simulink model "Crazyflie_CL_NL_Model"  (R2024a)
settings: Solver=ode23  StartTime=0.0  StopTime=Tend  FixedStep=dt  MaxStep=0.01  RelTol=1e-4
values from neighbouring files (symbols this model uses):
  ATTITUDE_RATE = 500    [crazyflie_Parameters.m]
  b = 1e-9    (= 1e-09)    [crazyflie_Parameters.m]
  cutoff_freq = 80    [crazyflie_Parameters.m]
  dt = 1/ATTITUDE_RATE    (= 0.002)    [crazyflie_Parameters.m]
  eta_eq0 = [0;0;0]    [Equilibrium_point.m]
  eta_init = eta_eq0    [Equilibrium_point.m]
  grav = 9.81    [crazyflie_Parameters.m]
  haero = 0    [crazyflie_Parameters.m]
  Jxx = rho_x_y*a_side*height*(a_side^2+height^2)/12    [crazyflie_Parameters.m]
  Jyy = rho_x_y*a_side*height*(a_side^2+height^2)/12    [crazyflie_Parameters.m]
  Jzz = rho_z*a_side^4/6    [crazyflie_Parameters.m]
  K = blkdiag(Kroll,Kpitch,Kyaw)*[1 0 0 0 0 0 ... (first row only)    [Basic_Classical_FR_control_design.m]
  kconst = 1.95e-8    (= 1.95e-08)    [crazyflie_Parameters.m]
  L = sqrt(a_side^2+a_side^2)/2    [crazyflie_Parameters.m]
  masse = 29e-3    (= 0.029)    [crazyflie_Parameters.m]
  MAXINT16 = 2^16-1    (= 65535)    [crazyflie_Parameters.m]
  Mc2u = [1  -0.5  0.5 -1 ... (first row only)    [crazyflie_Parameters.m]
  muxy = 0.4*masse    (= 0.0116)    [crazyflie_Parameters.m]
  muz = 5e-2    (= 0.05)    [crazyflie_Parameters.m]
  p0 = 280.93    [crazyflie_Parameters.m]
  p1 = 719.86    [crazyflie_Parameters.m]
  p2 = -15.689    [crazyflie_Parameters.m]
  p3 = 0.19157    [crazyflie_Parameters.m]
  p4 = -0.00082934    [crazyflie_Parameters.m]
  pdot_init = pdot_eq0    [Equilibrium_point.m]
  pitchSP = 2    [Equilibrium_point.m]
  pitchSPtime = 3    [Equilibrium_point.m]
  rollSP = 4    [Equilibrium_point.m]
  rollSPtime = 2.5    [Equilibrium_point.m]
  thurstSP = Tc    [Equilibrium_point.m]
  up = inpts(3)    [Equilibrium_point.m]    (also in mi_dron_film.m = R*[0;0;1])
  ur = inpts(2)    [Equilibrium_point.m]
  uy = inpts(4)    [Equilibrium_point.m]
  w_eq0 = [0;0;0]    [Equilibrium_point.m]
  w_init = w_eq0    [Equilibrium_point.m]
  yawSP = -3    [Equilibrium_point.m]
  yawSPtime = 2.1    [Equilibrium_point.m]
libraries: dspfdesign x6, cstblocks x1
settings Model: Creator=JB255047  LastModifiedBy=anton
settings SolverCC: AlgebraicLoopSolver=TrustRegion  DecoupledContinuousIntegration=on
settings DataIOCC: LimitDataPoints=on  SaveOutput=off  SignalLogging=off  DSMLogging=off  SaveTime=off
settings OptimizationCC: ExpressionDepthLimit=2147483647  LifeSpan=1
settings DebuggingCC: UnderspecifiedInitializationDetection=Classic  MergeDetectMultiDrivingBlocksExec=none  MultiTaskDSMMsg=none  FcnCallInpInsideContextMsg=warning  UnconnectedInputMsg=warning  UnconnectedOutputMsg=warning  UnconnectedLineMsg=warning  AllowSymbolicDim=off  StateNameClashWarn=warning  StrictBusMsg=ErrorOnBusTreatedAsVector  SFUnexpectedBacktrackingDiag=warning  SFNoUnconditionalDefaultTransitionDiag=warning  SFExecutionAtInitializationDiag=none  ArithmeticOperatorsInVariantConditions=warning
settings ModelReferenceCC: UpdateModelReferenceTargets=IfOutOfDate  EnableRefExpFcnMdlSchedulingChecks=on
settings SFSimCC: SFSimEcho=off  SimUseLocalCustomCode=off  CustomCodeUndefinedFunction=UseInterfaceOnly
settings RTWCC: RTWUseLocalCustomCode=off  GPUComputeCapability=3.5  DLArmComputeVersion=19.05
settings CodeAppCC: StateflowObjectComments=on
settings GRTTargetCC: TargetLangStandard=C89/C90 (ANSI)  CombineOutputUpdateFcns=off  GRTInterface=on

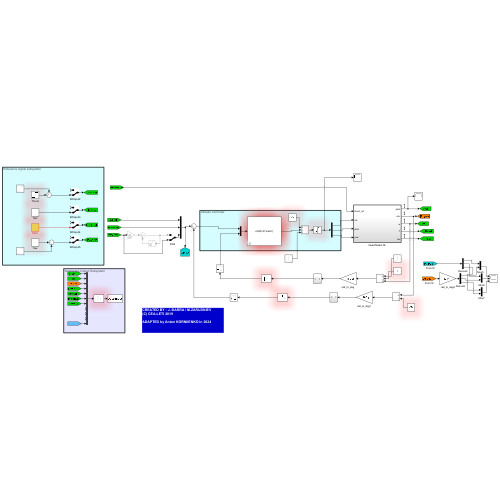
[thumbnail: Simulink's stored preview of the top-level diagram]
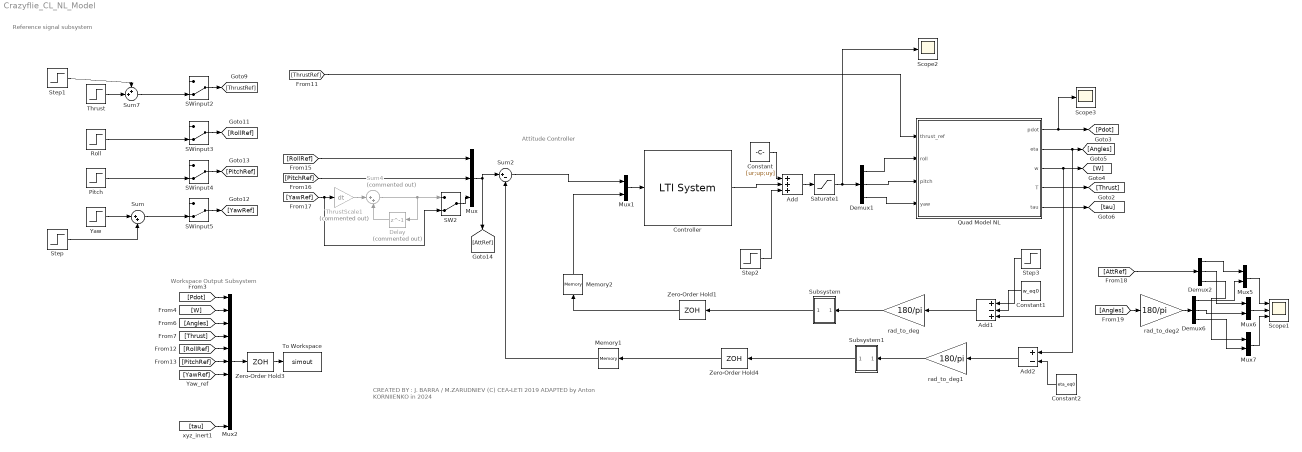
== system Crazyflie_CL_NL_Model ==
  note: CREATED BY : J. BARRA / M.ZARUDNIEV
      | (C) CEA-LETI 2019
      |
      | ADAPTED by Anton KORNIIENKO in 2024
  note: Workspace Output Subsystem
  note: Reference signal subsystem
  note: Attitude Controller
  Add : Sum  Inputs=+++
  Add1 : Sum  Inputs=+-+
  Add2 : Sum  Inputs=+-
  Constant : Constant  Value=[ur;up;uy]
  Constant1 : Constant  Value=w_eq0
  Constant2 : Constant  Value=eta_eq0
  Controller : cstblocks/LTI System  sys=c2d(K,dt,'tustin')  IC=[]  PadeOrder=0
  Delay : Delay  Commented=on  DelayLength=1  SampleTime=dt
  Demux1 : Demux  Outputs=3
  Demux2 : Demux  Outputs=3
  Demux6 : Demux  Outputs=3
  Memory1 : Memory
  Memory2 : Memory
  Mux : Mux  Inputs=3
  Mux{1,5..7} (4 alike) : Mux  Inputs=2
  Mux2 : Mux  Inputs=11
  Pitch : Step  Time=pitchSPtime  Before=up  After=pitchSP  SampleTime=0
  Quad Model NL : Subsystem  TreatAsAtomicUnit=on
  Roll : Step  Time=rollSPtime  Before=ur  After=rollSP  SampleTime=0
  SW2 : ManualSwitch  CurrentSetting=0
  SWinput{2..5} (4 alike) : ManualSwitch  CurrentSetting=0
  Saturate1 : Saturate  UpperLimit=MAXINT16/2-1  LowerLimit=-MAXINT16/2
  Scope1 : Scope  NumInputPorts=3
  Scope2 : Scope
  Scope3 : Scope
  Step : Step  Time=6.2  After=0  SampleTime=0
  Step1 : Step  Time=5  After=10000  SampleTime=0
  Step2 : Step  Time=7  After=-1000  SampleTime=0
  Step3 : Step  Time=14  SampleTime=0
  Subsystem : Subsystem
  Subsystem1 : Subsystem
  Sum : Sum  Inputs=|++
  Sum2 : Sum  Inputs=|+-
  Sum4 : Sum  Commented=on  Inputs=|++
  Sum7 : Sum  Inputs=++|
  Thrust : Step  Time=0  After=thurstSP  SampleTime=0
  ThrustScale1 : Gain  Commented=on  Gain=dt
  To Workspace : ToWorkspace  VariableName=simout  SaveFormat=Timeseries  SampleTime=-1
  Yaw : Step  Time=yawSPtime  Before=uy  After=yawSP  SampleTime=0
  Zero-Order Hold1 : ZeroOrderHold  SampleTime=1/ATTITUDE_RATE
  Zero-Order Hold3 : ZeroOrderHold  SampleTime=dt
  Zero-Order Hold4 : ZeroOrderHold  SampleTime=1/ATTITUDE_RATE
  rad_to_deg : Gain  Gain=180/pi
  rad_to_deg1 : Gain  Gain=180/pi
  rad_to_deg2 : Gain  Gain=180/pi
  wires:
  Sum2/1 -> Mux1/1
  Mux/1 -> Sum2/1, [AttRef]
  [ThrustRef] -> Quad Model NL/1(thrust_ref)
  Quad Model NL/3(w) -> Add1/3, [W]
  Mux2/1 -> Zero-Order Hold3/1
  Zero-Order Hold3/1 -> To Workspace/1
  [RollRef] -> Mux2/5
  [Pdot] -> Mux2/1
  [W] -> Mux2/2
  SWinput2/1 -> [ThrustRef]
  SWinput3/1 -> [RollRef]
  SWinput4/1 -> [PitchRef]
  SWinput5/1 -> [YawRef]
  Delay/1 -> Sum4/2
  [YawRef] -> SW2/2, ThrustScale1/1
  ThrustScale1/1 -> Sum4/1
  Sum4/1 -> SW2/1, Delay/1
  [PitchRef] -> Mux/2
  [RollRef] -> Mux/1
  Zero-Order Hold1/1 -> Memory2/1
  Zero-Order Hold4/1 -> Memory1/1
  Quad Model NL/2("eta ") -> Add2/1, [Angles]
  Memory1/1 -> Sum2/2
  Demux2/2 -> Mux6/1
  Demux6/2 -> Mux6/2
  Mux7/1 -> Scope1/3
  Mux6/1 -> Scope1/2
  Mux5/1 -> Scope1/1
  Demux2/3 -> Mux7/1
  Demux6/3 -> Mux7/2
  [AttRef] -> Demux2/1
  Demux6/1 -> Mux5/2
  Demux2/1 -> Mux5/1
  [Angles] -> rad_to_deg2/1
  SW2/1 -> Mux/3
  Roll/1 -> SWinput3/2
  Pitch/1 -> SWinput4/2
  Yaw/1 -> Sum/1
  Sum/1 -> SWinput5/2
  Step/1 -> Sum/2
  Quad Model NL/1(pdot) -> Scope3/1, [Pdot]
  Sum7/1 -> SWinput2/2
  Thrust/1 -> Sum7/2
  Step1/1 -> Sum7/1
  [Angles] -> Mux2/3
  [Thrust] -> Mux2/4
  [PitchRef] -> Mux2/6
  [YawRef] -> Mux2/7
  Quad Model NL/4(T) -> [Thrust]
  Quad Model NL/5(tau) -> [tau]
  [tau] -> Mux2/11
  rad_to_deg1/1 -> Subsystem1/1(In1)
  rad_to_deg/1 -> Subsystem/1(In1)
  Subsystem/1(Out1) -> Zero-Order Hold1/1
  Subsystem1/1(Out1) -> Zero-Order Hold4/1
  rad_to_deg2/1 -> Demux6/1
  Memory2/1 -> Mux1/2
  Mux1/1 -> Controller/1
  Demux1/1 -> Quad Model NL/2(roll)
  Demux1/2 -> Quad Model NL/3(pitch)
  Demux1/3 -> Quad Model NL/4(yaw)
  Add/1 -> Saturate1/1
  Constant/1 -> Add/1
  Controller/1 -> Add/2
  Saturate1/1 -> Scope2/1, Demux1/1
  Add1/1 -> rad_to_deg/1
  Add2/1 -> rad_to_deg1/1
  Constant1/1 -> Add1/2
  Constant2/1 -> Add2/2
  Step2/1 -> Add/3
  Step3/1 -> Add1/1

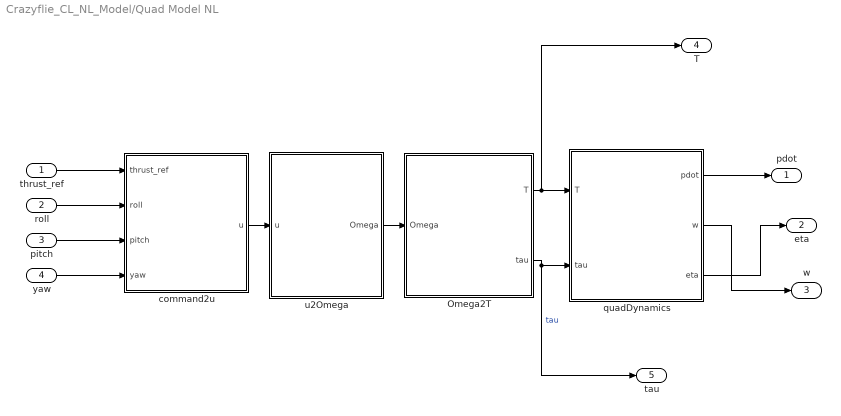
== system Crazyflie_CL_NL_Model/Quad Model NL ==
  thrust_ref : Inport
  roll : Inport  Port=2
  pitch : Inport  Port=3
  yaw : Inport  Port=4
  Omega2T : Subsystem  InitFcn=Omega=zeros(4,1);
  command2u : Subsystem  InitFcn=u=zeros(4,1);
  "quadDynamics " : Subsystem
  u2Omega : Subsystem
  pdot : Outport  VectorParamsAs1DForOutWhenUnconnected=off
  "eta " : Outport  Port=2  VectorParamsAs1DForOutWhenUnconnected=off
  w : Outport  Port=3  VectorParamsAs1DForOutWhenUnconnected=off
  T : Outport  Port=4  VectorParamsAs1DForOutWhenUnconnected=off
  tau : Outport  Port=5  VectorParamsAs1DForOutWhenUnconnected=off
  wires:
  "quadDynamics "/2(w) -> w/1
  "quadDynamics "/1(pdot) -> pdot/1
  "quadDynamics "/3(eta) -> "eta "/1
  Omega2T/1(T) -> "quadDynamics "/1(T), T/1
  thrust_ref/1 -> command2u/1(thrust_ref)
  roll/1 -> command2u/2(roll)
  pitch/1 -> command2u/3(pitch)
  yaw/1 -> command2u/4(yaw)
  Omega2T/2(tau) -> "quadDynamics "/2(tau), tau/1  "tau"
  u2Omega/1(Omega) -> Omega2T/1(Omega)
  command2u/1(u) -> u2Omega/1(u)

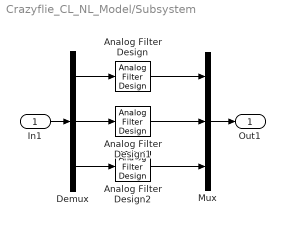
== system Crazyflie_CL_NL_Model/Subsystem ==
  In1 : Inport
  Analog Filter Design : dspfdesign/Analog Filter Design  method=Butterworth  filttype=Lowpass  N=2  Wlo=2*pi*cutoff_freq  Whi=80  Rp=2  Rs=40
  Analog Filter Design1 : dspfdesign/Analog Filter Design  method=Butterworth  filttype=Lowpass  N=2  Wlo=2*pi*cutoff_freq  Whi=80  Rp=2  Rs=40
  Analog Filter Design2 : dspfdesign/Analog Filter Design  method=Butterworth  filttype=Lowpass  N=2  Wlo=2*pi*cutoff_freq  Whi=80  Rp=2  Rs=40
  Demux : Demux  Outputs=3
  Mux : Mux  Inputs=3
  Out1 : Outport  VectorParamsAs1DForOutWhenUnconnected=off
  wires:
  In1/1 -> Demux/1
  Demux/1 -> Analog Filter Design/1
  Demux/2 -> Analog Filter Design1/1
  Demux/3 -> Analog Filter Design2/1
  Analog Filter Design1/1 -> Mux/2
  Analog Filter Design/1 -> Mux/1
  Analog Filter Design2/1 -> Mux/3
  Mux/1 -> Out1/1

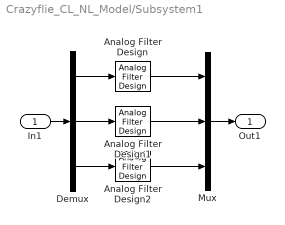
== system Crazyflie_CL_NL_Model/Subsystem1 ==
  In1 : Inport
  Analog Filter Design : dspfdesign/Analog Filter Design  method=Butterworth  filttype=Lowpass  N=2  Wlo=2*pi*cutoff_freq  Whi=80  Rp=2  Rs=40
  Analog Filter Design1 : dspfdesign/Analog Filter Design  method=Butterworth  filttype=Lowpass  N=2  Wlo=2*pi*cutoff_freq  Whi=80  Rp=2  Rs=40
  Analog Filter Design2 : dspfdesign/Analog Filter Design  method=Butterworth  filttype=Lowpass  N=2  Wlo=2*pi*cutoff_freq  Whi=80  Rp=2  Rs=40
  Demux : Demux  Outputs=3
  Mux : Mux  Inputs=3
  Out1 : Outport  VectorParamsAs1DForOutWhenUnconnected=off
  wires:
  In1/1 -> Demux/1
  Demux/1 -> Analog Filter Design/1
  Demux/2 -> Analog Filter Design1/1
  Demux/3 -> Analog Filter Design2/1
  Analog Filter Design1/1 -> Mux/2
  Analog Filter Design/1 -> Mux/1
  Analog Filter Design2/1 -> Mux/3
  Mux/1 -> Out1/1

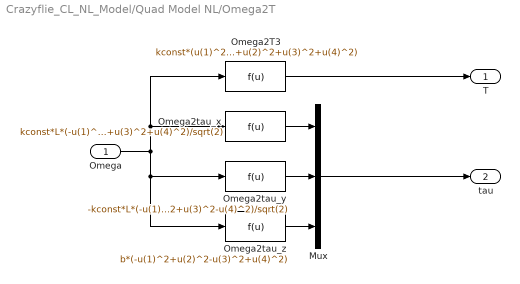
== system Crazyflie_CL_NL_Model/Quad Model NL/Omega2T ==
  Omega : Inport  PortDimensions=4
  Mux : Mux  Inputs=3
  Omega2T3 : Fcn  Expr=kconst*(u(1)^2+u(2)^2+u(3)^2+u(4)^2)
  Omega2tau_x : Fcn  Expr=kconst*L*(-u(1)^2-u(2)^2+u(3)^2+u(4)^2)/sqrt(2)
  Omega2tau_y : Fcn  Expr=-kconst*L*(-u(1)^2+u(2)^2+u(3)^2-u(4)^2)/sqrt(2)
  Omega2tau_z : Fcn  Expr=b*(-u(1)^2+u(2)^2-u(3)^2+u(4)^2)
  T : Outport  VectorParamsAs1DForOutWhenUnconnected=off
  tau : Outport  Port=2  VectorParamsAs1DForOutWhenUnconnected=off
  wires:
  Omega/1 -> Omega2T3/1, Omega2tau_x/1, Omega2tau_y/1, Omega2tau_z/1
  Omega2tau_z/1 -> Mux/3
  Omega2tau_x/1 -> Mux/1
  Omega2tau_y/1 -> Mux/2
  Mux/1 -> tau/1
  Omega2T3/1 -> T/1

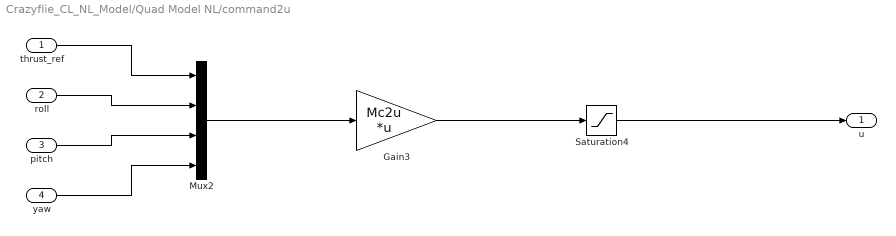
== system Crazyflie_CL_NL_Model/Quad Model NL/command2u ==
  thrust_ref : Inport
  roll : Inport  Port=2
  pitch : Inport  Port=3
  yaw : Inport  Port=4
  Gain3 : Gain  Gain=Mc2u  Multiplication=Matrix(K*u)
  Mux2 : Mux
  Saturation4 : Saturate  UpperLimit=MAXINT16  LowerLimit=0  LinearizeAsGain=off  ZeroCross=off
  u : Outport  VectorParamsAs1DForOutWhenUnconnected=off
  wires:
  thrust_ref/1 -> Mux2/1
  roll/1 -> Mux2/2
  pitch/1 -> Mux2/3
  yaw/1 -> Mux2/4
  Mux2/1 -> Gain3/1
  Gain3/1 -> Saturation4/1
  Saturation4/1 -> u/1

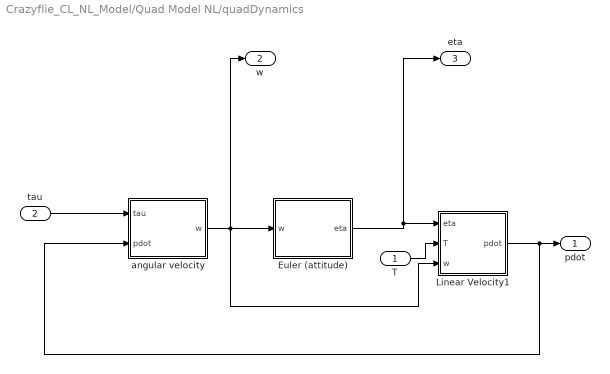
== system Crazyflie_CL_NL_Model/Quad Model NL/quadDynamics  ==
  T : Inport
  tau : Inport  Port=2
  "Euler (attitude) " : Subsystem
  Linear Velocity1 : Subsystem
  angular velocity : Subsystem
  pdot : Outport  PortDimensions=3  VectorParamsAs1DForOutWhenUnconnected=off
  w : Outport  Port=2  PortDimensions=3  VectorParamsAs1DForOutWhenUnconnected=off
  eta : Outport  Port=3  PortDimensions=3  VectorParamsAs1DForOutWhenUnconnected=off
  wires:
  T/1 -> Linear Velocity1/2(T)
  Linear Velocity1/1(pdot) -> angular velocity/2(pdot), pdot/1
  tau/1 -> angular velocity/1(tau)
  "Euler (attitude) "/1("eta ") -> eta/1, Linear Velocity1/1(eta)
  angular velocity/1(w) -> Linear Velocity1/3(w), w/1, "Euler (attitude) "/1(w)

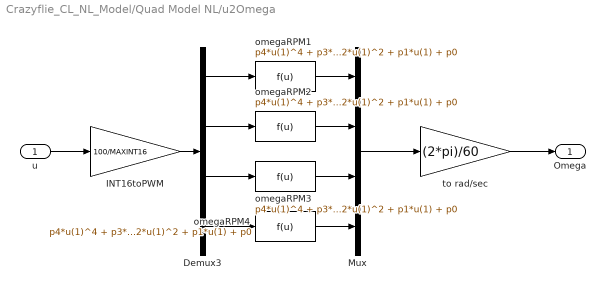
== system Crazyflie_CL_NL_Model/Quad Model NL/u2Omega ==
  u : Inport  PortDimensions=4
  Demux3 : Demux
  INT16toPWM : Gain  Gain=100/MAXINT16
  Mux : Mux
  omegaRPM{1..4} (4 alike) : Fcn  Expr=p4*u(1)^4 + p3*u(1)^3 + p2*u(1)^2 + p1*u(1) + p0
  to rad/sec : Gain  Gain=(2*pi)/60
  Omega : Outport  PortDimensions=4  VectorParamsAs1DForOutWhenUnconnected=off
  wires:
  u/1 -> INT16toPWM/1
  Mux/1 -> to rad/sec/1
  INT16toPWM/1 -> Demux3/1
  omegaRPM1/1 -> Mux/1
  Demux3/1 -> omegaRPM1/1
  Demux3/2 -> omegaRPM2/1
  omegaRPM2/1 -> Mux/2
  Demux3/3 -> omegaRPM3/1
  Demux3/4 -> omegaRPM4/1
  omegaRPM3/1 -> Mux/3
  omegaRPM4/1 -> Mux/4
  to rad/sec/1 -> Omega/1

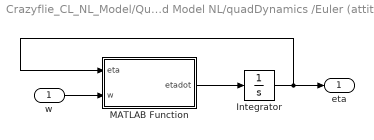
== system Crazyflie_CL_NL_Model/Quad Model NL/quadDynamics /Euler (attitude)  ==
  w : Inport  OutDataTypeStr=double
  Integrator : Integrator  InitialCondition=eta_init
  MATLAB Function : MATLAB Function  TreatAsAtomicUnit=on
  "eta " : Outport  VectorParamsAs1DForOutWhenUnconnected=off
  wires:
  Integrator/1 -> MATLAB Function/1(eta), "eta "/1
  w/1 -> MATLAB Function/2(w)
  MATLAB Function/1(etadot) -> Integrator/1

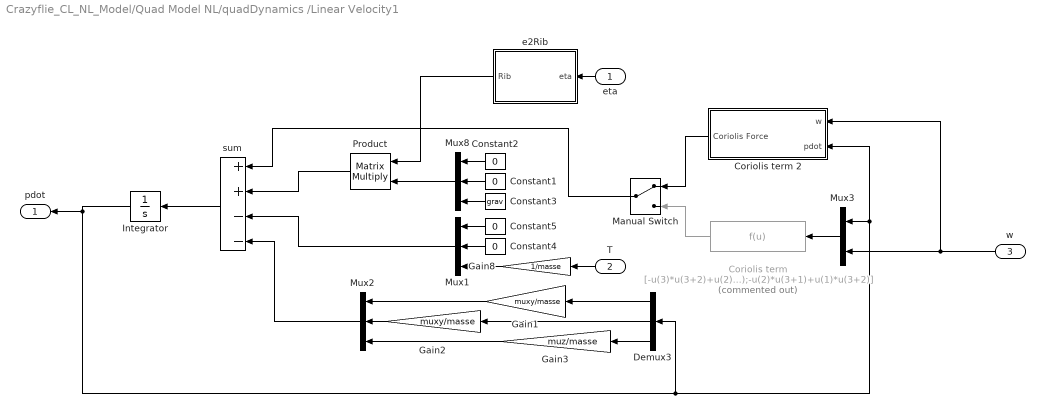
== system Crazyflie_CL_NL_Model/Quad Model NL/quadDynamics /Linear Velocity1 ==
  eta : Inport
  T : Inport  Port=2
  w : Inport  Port=3
  Constant{1..2,4..5} (4 alike) : Constant  Value=0
  Constant3 : Constant  Value=grav
  Coriolis term : Fcn  Commented=on  Expr=[-u(3)*u(3+2)+u(2)*u(3+3);-u(1)*u(3+3)+u(3)*u(3+1);-u(2)*u(3+1)+u(1)*u(3+2)]
  Coriolis term 2 : Subsystem
  Demux3 : Demux  Outputs=3
  Gain1 : Gain  Gain=muxy/masse
  Gain2 : Gain  Gain=muxy/masse
  Gain3 : Gain  Gain=muz/masse
  Gain8 : Gain  Gain=1/masse
  Integrator : Integrator  InitialCondition=pdot_init
  Manual Switch : ManualSwitch
  Mux1 : Mux  Inputs=3
  Mux2 : Mux  Inputs=3
  Mux3 : Mux  Inputs=2
  Mux8 : Mux  Inputs=3
  Product : Product  Multiplication=Matrix(*)  InputSameDT=on  SaturateOnIntegerOverflow=on  OutDataTypeStr=Inherit: Same as first input
  e2Rib : Subsystem
  sum : Sum  Inputs=++--
  pdot : Outport  PortDimensions=3  VectorParamsAs1DForOutWhenUnconnected=off
  wires:
  Constant1/1 -> Mux8/2
  Integrator/1 -> Demux3/1, Coriolis term 2/2(pdot), Mux3/1, pdot/1
  Constant4/1 -> Mux1/2
  T/1 -> Gain8/1
  Constant5/1 -> Mux1/1
  Gain1/1 -> Mux2/1
  Gain3/1 -> Mux2/3
  Gain8/1 -> Mux1/3
  Demux3/3 -> Gain3/1
  Gain2/1 -> Mux2/2
  eta/1 -> e2Rib/1(eta)
  Constant2/1 -> Mux8/1
  Mux2/1 -> sum/4
  sum/1 -> Integrator/1
  Mux1/1 -> sum/3
  Product/1 -> sum/2
  Constant3/1 -> Mux8/3
  Mux8/1 -> Product/2
  Demux3/1 -> Gain1/1
  Demux3/2 -> Gain2/1
  e2Rib/1(Rib) -> Product/1
  w/1 -> Coriolis term 2/1(w), Mux3/2
  Mux3/1 -> Coriolis term/1
  Coriolis term/1 -> Manual Switch/2
  Manual Switch/1 -> sum/1
  Coriolis term 2/1(Coriolis Force) -> Manual Switch/1

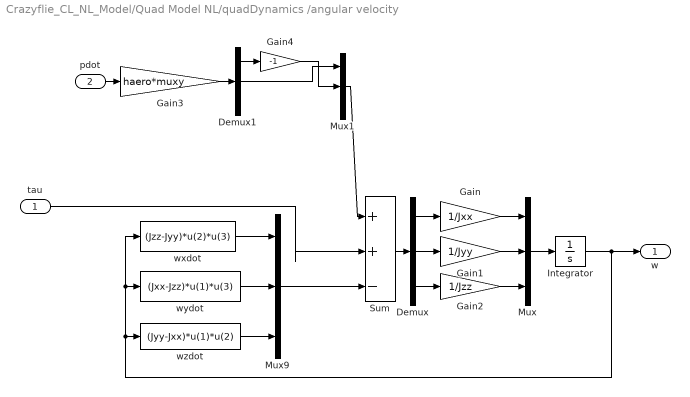
== system Crazyflie_CL_NL_Model/Quad Model NL/quadDynamics /angular velocity ==
  tau : Inport
  pdot : Inport  Port=2
  Demux : Demux  Outputs=3
  Demux1 : Demux  Outputs=3
  Gain : Gain  Gain=1/Jxx
  Gain1 : Gain  Gain=1/Jyy
  Gain2 : Gain  Gain=1/Jzz
  Gain3 : Gain  Gain=haero*muxy
  Gain4 : Gain  Gain=-1
  Integrator : Integrator  InitialCondition=w_init
  Mux : Mux  Inputs=3
  Mux1 : Mux  Inputs=3
  Mux9 : Mux  Inputs=3
  Sum : Sum  Inputs=|++-
  wxdot : Fcn  Expr=(Jzz-Jyy)*u(2)*u(3)
  wydot : Fcn  Expr=(Jxx-Jzz)*u(1)*u(3)
  wzdot : Fcn  Expr=(Jyy-Jxx)*u(1)*u(2)
  w : Outport  PortDimensions=3  VectorParamsAs1DForOutWhenUnconnected=off
  wires:
  wzdot/1 -> Mux9/3
  Sum/1 -> Demux/1
  Demux/1 -> Gain/1
  Demux/2 -> Gain1/1
  Demux/3 -> Gain2/1
  Gain/1 -> Mux/1
  Gain1/1 -> Mux/2
  Gain2/1 -> Mux/3
  Mux/1 -> Integrator/1
  Integrator/1 -> w/1, wzdot/1, wydot/1, wxdot/1
  wydot/1 -> Mux9/2
  wxdot/1 -> Mux9/1
  pdot/1 -> Gain3/1
  Gain3/1 -> Demux1/1
  Demux1/2 -> Mux1/1
  Mux1/1 -> Sum/1
  Demux1/1 -> Gain4/1
  Gain4/1 -> Mux1/2
  tau/1 -> Sum/2
  Mux9/1 -> Sum/3

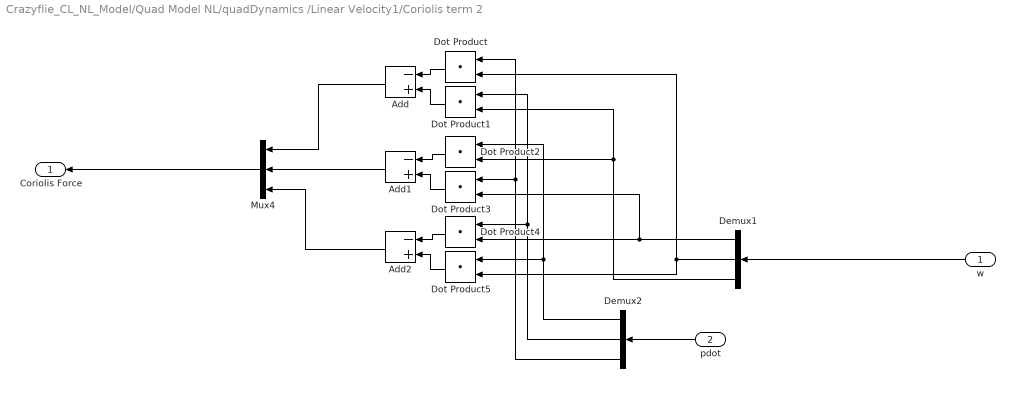
== system Crazyflie_CL_NL_Model/Quad Model NL/quadDynamics /Linear Velocity1/Coriolis term 2 ==
  w : Inport
  pdot : Inport  Port=2
  Add : Sum  Inputs=-+
  Add1 : Sum  Inputs=-+
  Add2 : Sum  Inputs=-+
  Demux1 : Demux  Outputs=3
  Demux2 : Demux  Outputs=3
  Dot Product{,1..5} (6 alike) : DotProduct  OutDataTypeStr=Inherit: Inherit via internal rule
  Mux4 : Mux  Inputs=3
  Coriolis Force : Outport
  wires:
  Demux2/1 -> Dot Product5/1, Dot Product2/1
  Add/1 -> Mux4/1
  Dot Product4/1 -> Add2/1
  Demux1/1 -> Dot Product4/2, Dot Product3/2
  Dot Product1/1 -> Add/2
  Demux1/3 -> Dot Product2/2, Dot Product1/2
  Add1/1 -> Mux4/2
  Dot Product2/1 -> Add1/1
  Demux2/3 -> Dot Product3/1, Dot Product/1
  Demux1/2 -> Dot Product5/2, Dot Product/2
  Dot Product3/1 -> Add1/2
  Dot Product/1 -> Add/1
  Dot Product5/1 -> Add2/2
  Demux2/2 -> Dot Product4/1, Dot Product1/1
  Add2/1 -> Mux4/3
  w/1 -> Demux1/1
  pdot/1 -> Demux2/1
  Mux4/1 -> Coriolis Force/1

== system Crazyflie_CL_NL_Model/Quad Model NL/quadDynamics /Linear Velocity1/e2Rib ==
  eta : Inport
  MATLAB Function : MATLAB Function  TreatAsAtomicUnit=on
  Rib : Outport  VectorParamsAs1DForOutWhenUnconnected=off
  wires:
  eta/1 -> MATLAB Function/1(eta)
  MATLAB Function/1(R_ib) -> Rib/1

== matlab function Crazyflie_CL_NL_Model/Quad Model NL/quadDynamics /Linear Velocity1/e2Rib/MATLAB Function ==
  data: eta input; R_ib output
function R_ib  = eR_ib(eta)
%%
%% Author               : Jérémy Barra
%% Organization         : CEA/LETI
%% COPYRIGHT            : CEA
%%                      :
%% Short description    : Return the rotation matrix from the inertial to
%%                      : the body frame
%%                      :
%% Inputs               
%   Attitude euler angles: eta=[phi; theta; psi]
%% Outputs               
%   Rotation matrix from inertial to body frame: R_ib
%% Remarks
%   1 dimensional vectors are given in columns 
%%
cphi=cos(eta(1));
sphi=sin(eta(1));
ctheta=cos(eta(2));
stheta=sin(eta(2));
cpsi=cos(eta(3));
spsi=sin(eta(3));

R_ib=[ctheta*cpsi spsi*ctheta -stheta;
    cpsi*stheta*sphi-spsi*cphi spsi*stheta*sphi+cphi*cpsi ctheta*sphi;
    cpsi*stheta*cphi+sphi*spsi spsi*stheta*cphi-cpsi*sphi cphi*ctheta];

%R_ib=[0 0 -stheta;
%      0 0 ctheta*sphi;
%      0 0 cphi*ctheta];

end

== matlab function Crazyflie_CL_NL_Model/Quad Model NL/quadDynamics /Euler (attitude) /MATLAB Function ==
  data: eta input; etadot output; w input

function etadot = fcn(eta,w)
etadot=[w(1)+sin(eta(1))*tan(eta(2))*w(2)+cos(eta(1))*tan(eta(2))*w(3);
    cos(eta(1))*w(2)-sin(eta(1))*w(3);
    (sin(eta(1))/cos(eta(2)))*w(2)+(cos(eta(1))/cos(eta(2)))*w(3)];
end
